simulink model "PHIL_testing"  (R2023b)
settings: Solver=ode4  StartTime=0.0  StopTime=inf  FixedStep=Ts  RelTol=1e-3
PostLoadFcn:
  | init;
InitFcn:
  | init;
values from neighbouring files (symbols this model uses):
  CURRENT_INPUT_OFFSET_PHA = 0    [init.m]
  CURRENT_INPUT_OFFSET_PHB = 0    [init.m]
  CURRENT_INPUT_OFFSET_PHC = 0    [init.m]
  CURRENT_INPUT_SCALE_PHA = 30    [init.m]
  CURRENT_INPUT_SCALE_PHB = 30    [init.m]
  CURRENT_INPUT_SCALE_PHC = 30    [init.m]
  ENABLE_PHA = 1    [init.m]
  ENABLE_PHB = 1    [init.m]
  ENABLE_PHC = 1    [init.m]
  FNOM = 60.0    (= 60)    [init.m]
  FREQUENCY = 60.0    (= 60)    [init.m]
  FREQUENCY_MAX_LIMIT = 66.0    (= 66)    [init.m]
  FREQUENCY_MIN_LIMIT = 56.0    (= 56)    [init.m]
  FRT_CONDITION = [1 1 1 0 ]    [init.m]
  FRT_END_TIMING = [0.2 0.3 0.4 0.5]    [init.m]
  FRT_START_TIMING = [0.1 0.2 0.3 0.4]    [init.m]
  FRT_VALUES = [59.0 56.0 55.0 33.0]    [init.m]
  MODE = 1    [init.m]
  PCRT_CONDITION = [ 0    1     0     2     0     3      0      4      0      4      0   ]    [init.m]
  PCRT_END_TIMING = [30.0 30.32 60.32 60.64 90.64 90.96 120.96 175.96 205.96 260.96 290.96]    [init.m]
  PCRT_START_TIMING = [ 0.0 30.0  30.32 60.32 60.64 90.64  90.96 120.96 175.96 205.96 260.96]    [init.m]
  PCRT_VALUES = [ 0.0 60.0   0.0  60.0   0.0  60.0    0.0   20.0    0.0  340.0    0.0 ]    [init.m]
  PHASE = [0.0 -120.0 120.0]    [init.m]
  PHNOM = [0 -120 120]    [init.m]
  Pnom = 5e3    (= 5000)    [init.m]
  RMS_ENABLE = 0    [init.m]
  ROCOF_ENABLE = 0    [init.m]
  ROCOF_INIT = 60    [init.m]
  ROCOF_VALUE = 3    [init.m]
  ROCOM_ENABLE = 1    [init.m]
  ROCOM_END_TIME = 100    [init.m]
  ROCOM_INIT = 1    [init.m]
  ROCOM_START_TIME = 0    [init.m]
  ROCOM_VALUE = 13.8    [init.m]
  Srated = 5e3    (= 5000)    [init.m]
  Ts = 40e-6    (= 4e-05)    [init.m]
  VNOM = 1.0    (= 1)    [init.m]
  VOLT_INPUT_OFFSET_PHA = 0    [init.m]
  VOLT_INPUT_OFFSET_PHB = 0    [init.m]
  VOLT_INPUT_OFFSET_PHC = 0    [init.m]
  VOLT_INPUT_SCALE_PHA = 100    [init.m]
  VOLT_INPUT_SCALE_PHB = 100    [init.m]
  VOLT_INPUT_SCALE_PHC = 100    [init.m]
  VOLT_OUTPUT_SCALE_PHA = 5.6    [init.m]
  VOLT_OUTPUT_SCALE_PHB = 5.6    [init.m]
  VOLT_OUTPUT_SCALE_PHC = 5.6    [init.m]
  VOLTAGE = [1.0 1.0 1.0]    [init.m]
  VOLTAGE_MAX_LIMIT = 1.1    [init.m]
  VOLTAGE_MIN_LIMIT = 0.0    (= 0)    [init.m]
  VRT_CONDITION = [0 1 0 1 0 1 0 1 -1 -1 -1 -1 -1 -1 -1 -1 -1 -1 -1 -1]+1    [init.m]
  VRT_END_TIMING = [0.2 0.3 0.4 0.5 0.6 0.7 0.8 0.9 1 1.1 1.2 1.3 1.4 1.5 1.6 1.7 1.8 1.9 2 2.1]    [init.m]
  VRT_PHA_ENABLE = 0    [init.m]
  VRT_PHB_ENABLE = 0    [init.m]
  VRT_PHC_ENABLE = 0    [init.m]
  VRT_START_TIMING = [0.1 0.2 0.3 0.4 0.5 0.6 0.7 0.8 0.9 1 0.1 0.2 0.3 0.4 0.5 0.6 0.7 0.8 0.9 1]    [init.m]
  VRT_VALUES = [1.2 0.94 0 0.5 0.7 0.88 0.94 0.88 0.94 1.1 1.2 0.94 0 0.5 0.7 0.88 0.94 0.88 0.94 1.1]    [init.m]
  WAV_ENABLE = 1    [init.m]
undefined symbols (not defined in the file or in its folder): another_event_name, DiscIntNeverNeededParam, EX, magnitude, my_event_name, TE0741_4, TwoSSS_AIO_CPWM
libraries: simulink x14, rtlab x6, simulink_extras x6, spsRMSLib x6, rtio_opalrt_common x4, eePowerMeasurement x3, rtio_opalrt_ml605ex1 x2, spsPLL3phLib x1, spspowerguiLib x1
(part 2 of 2)

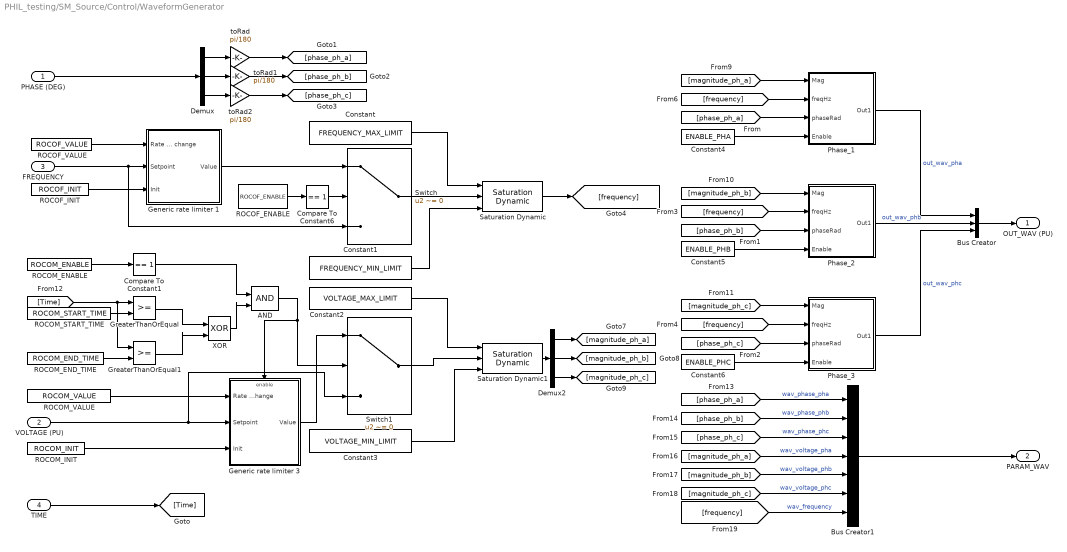
== system PHIL_testing/SM_Source/Control/WaveformGenerator ==
  PHASE (DEG) : Inport
  VOLTAGE (PU) : Inport  Port=2
  FREQUENCY : Inport  Port=3
  TIME : Inport  Port=4
  AND : Logic  IconShape=distinctive  AllPortsSameDT=off  OutDataTypeStr=boolean
  Bus Creator : BusCreator  Inputs=3
  Bus Creator1 : BusCreator  Inputs=7
  Compare To Constant1 : simulink/Logic and Bit Operations/Compare To Constant  relop===  const=1  OutDataTypeStr=boolean
  Compare To Constant6 : simulink/Logic and Bit Operations/Compare To Constant  relop===  const=1  OutDataTypeStr=boolean
  Constant : Constant  Value=FREQUENCY_MAX_LIMIT
  Constant1 : Constant  Value=FREQUENCY_MIN_LIMIT
  Constant2 : Constant  Value=VOLTAGE_MAX_LIMIT
  Constant3 : Constant  Value=VOLTAGE_MIN_LIMIT
  Constant4 : Constant  Value=ENABLE_PHA
  Constant5 : Constant  Value=ENABLE_PHB
  Constant6 : Constant  Value=ENABLE_PHC
  Demux : Demux  Outputs=3
  Demux2 : Demux  Outputs=3
  Generic rate limiter 1 : Subsystem
  Generic rate limiter 3 : Subsystem
  GreaterThanOrEqual : RelationalOperator  OutDataTypeStr=boolean  RndMeth=Simplest  InputSameDT=off
  GreaterThanOrEqual1 : RelationalOperator  OutDataTypeStr=boolean  RndMeth=Simplest  InputSameDT=off
  Phase_1 : Subsystem
  Phase_2 : Subsystem
  Phase_3 : Subsystem
  ROCOF_ENABLE : Constant  Value=ROCOF_ENABLE
  ROCOF_INIT : Constant  Value=ROCOF_INIT
  ROCOF_VALUE : Constant  Value=ROCOF_VALUE
  ROCOM_ENABLE : Constant  Value=ROCOM_ENABLE
  ROCOM_END_TIME : Constant  Value=ROCOM_END_TIME
  ROCOM_INIT : Constant  Value=ROCOM_INIT
  ROCOM_START_TIME : Constant  Value=ROCOM_START_TIME
  ROCOM_VALUE : Constant  Value=ROCOM_VALUE
  Saturation Dynamic : simulink/Discontinuities/Saturation Dynamic  OutMin=[]  OutMax=[]  OutDataTypeStr=Inherit: Same as second input  OutDataType=fixdt(1, 16)  OutScaling=2^-10  DoSatur=off
  Saturation Dynamic1 : simulink/Discontinuities/Saturation Dynamic  OutMin=[]  OutMax=[]  OutDataTypeStr=Inherit: Same as second input  OutDataType=fixdt(1, 16)  OutScaling=2^-10  DoSatur=off
  Switch : Switch  Criteria=u2 ~= 0  SaturateOnIntegerOverflow=off  InputSameDT=off
  Switch1 : Switch  Criteria=u2 ~= 0  SaturateOnIntegerOverflow=off  InputSameDT=off
  XOR : Logic  Operator=XOR  IconShape=distinctive  AllPortsSameDT=off  OutDataTypeStr=boolean
  toRad : Gain  Gain=pi/180
  toRad1 : Gain  Gain=pi/180
  toRad2 : Gain  Gain=pi/180
  OUT_WAV (PU) : Outport
  PARAM_WAV : Outport  Port=2
  wires:
  VOLTAGE (PU)/1 -> Generic rate limiter 3/2("Setpoint "), Switch1/3
  PHASE (DEG)/1 -> Demux/1
  Demux/1 -> toRad/1
  Demux/2 -> toRad1/1
  Demux/3 -> toRad2/1
  [phase_ph_a] -> Phase_1/3(phaseRad)
  [phase_ph_b] -> Phase_2/3(phaseRad)
  [phase_ph_c] -> Phase_3/3(phaseRad)
  Generic rate limiter 1/1(Value) -> Switch/1
  FREQUENCY/1 -> Switch/3, Generic rate limiter 1/2("Setpoint ")
  ROCOF_VALUE/1 -> Generic rate limiter 1/1(Rate of change)
  ROCOF_INIT/1 -> Generic rate limiter 1/3(Init)
  ROCOF_ENABLE/1 -> Compare To Constant6/1
  Compare To Constant6/1 -> Switch/2
  ROCOM_VALUE/1 -> Generic rate limiter 3/1(Rate of change)
  ROCOM_INIT/1 -> Generic rate limiter 3/3(Init)
  [frequency] -> Phase_1/2(freqHz)
  [frequency] -> Phase_2/2(freqHz)
  Demux2/1 -> [magnitude_ph_a]
  Demux2/2 -> [magnitude_ph_b]
  Demux2/3 -> [magnitude_ph_c]
  [magnitude_ph_a] -> Phase_1/1(Mag)
  [magnitude_ph_b] -> Phase_2/1(Mag)
  [magnitude_ph_c] -> Phase_3/1(Mag)
  [Time] -> GreaterThanOrEqual1/1, GreaterThanOrEqual/1
  ROCOM_START_TIME/1 -> GreaterThanOrEqual/2
  ROCOM_END_TIME/1 -> GreaterThanOrEqual1/2
  GreaterThanOrEqual/1 -> XOR/1
  GreaterThanOrEqual1/1 -> XOR/2
  Switch1/1 -> Saturation Dynamic1/2
  Generic rate limiter 3/1(Value) -> Switch1/1
  AND/1 -> Switch1/2, Generic rate limiter 3/Enable
  XOR/1 -> AND/2
  Compare To Constant1/1 -> AND/1
  ROCOM_ENABLE/1 -> Compare To Constant1/1
  Switch/1 -> Saturation Dynamic/2
  TIME/1 -> [Time]
  Phase_1/1(Out1) -> Bus Creator/1  "out_wav_pha"
  Phase_2/1(Out1) -> Bus Creator/2  "out_wav_phb"
  Phase_3/1(Out1) -> Bus Creator/3  "out_wav_phc"
  Bus Creator/1 -> OUT_WAV (PU)/1
  [phase_ph_a] -> Bus Creator1/1  "wav_phase_pha"
  [phase_ph_b] -> Bus Creator1/2  "wav_phase_phb"
  [phase_ph_c] -> Bus Creator1/3  "wav_phase_phc"
  [magnitude_ph_a] -> Bus Creator1/4  "wav_voltage_pha"
  [magnitude_ph_b] -> Bus Creator1/5  "wav_voltage_phb"
  [magnitude_ph_c] -> Bus Creator1/6  "wav_voltage_phc"
  [frequency] -> Bus Creator1/7  "wav_frequency"
  Bus Creator1/1 -> PARAM_WAV/1
  Saturation Dynamic/1 -> [frequency]
  Saturation Dynamic1/1 -> Demux2/1
  Constant/1 -> Saturation Dynamic/1
  Constant1/1 -> Saturation Dynamic/3
  Constant2/1 -> Saturation Dynamic1/1
  Constant3/1 -> Saturation Dynamic1/3
  toRad/1 -> [phase_ph_a]
  toRad1/1 -> [phase_ph_b]
  toRad2/1 -> [phase_ph_c]
  Constant4/1 -> Phase_1/4(Enable)
  Constant5/1 -> Phase_2/4(Enable)
  [frequency] -> Phase_3/2(freqHz)
  Constant6/1 -> Phase_3/4(Enable)

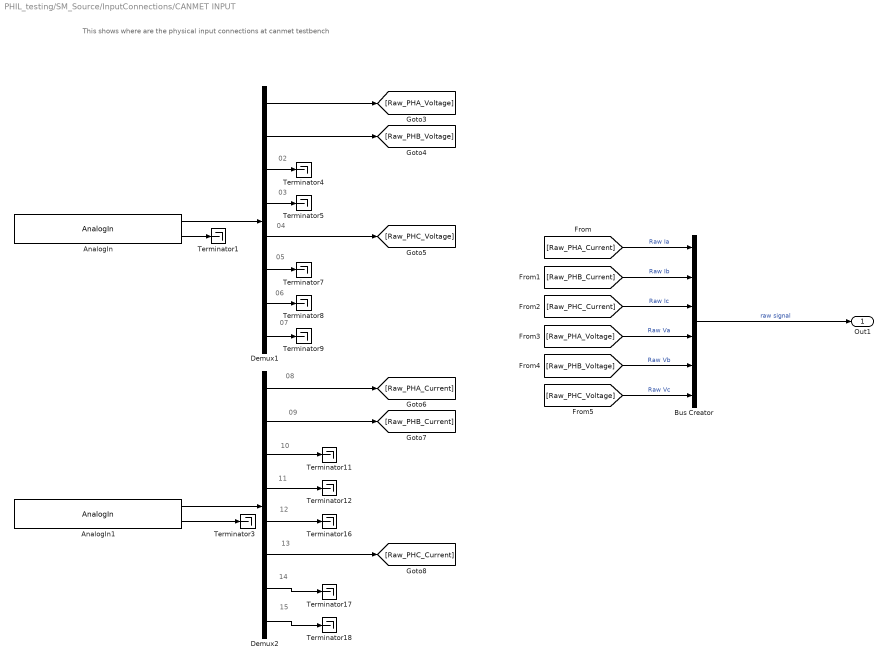
== system PHIL_testing/SM_Source/InputConnections/CANMET INPUT ==
  note: This shows where are the physical input connections at canmet testbench
  note: 10
  note: 08
  note: 03
  note: 04
  note: 15
  note: 12
  note: 09
  note: 06
  note: 11
  note: 07
  note: 05
  note: 02
  note: 13
  note: 14
  AnalogIn : rtio_opalrt_common/AnalogIn  CtrlName='OpCtrl'  portNb=7  FcnNos=Slot 6 Module A Subsection 1  size=16  maxcount=8  count=8  numchan=8  sampleTime=0
      settings: AttributesFormatString=%<CtrlName>  SourceProductName=RT-LAB I/O
  AnalogIn1 : rtio_opalrt_common/AnalogIn  CtrlName='OpCtrl'  portNb=8  FcnNos=Slot 6 Module A Subsection 2  size=16  maxcount=8  count=8  numchan=8  sampleTime=0
      settings: AttributesFormatString=%<CtrlName>  SourceProductName=RT-LAB I/O
  Bus Creator : BusCreator  Inputs=6
  Demux1 : Demux  Outputs=8
  Demux2 : Demux  Outputs=8
  Terminator{1,3..5,7..9,11..12,16..18} (12 alike) : Terminator
  Out1 : Outport  VectorParamsAs1DForOutWhenUnconnected=off
  wires:
  AnalogIn/2 -> Terminator1/1
  AnalogIn1/2 -> Terminator3/1
  AnalogIn/1 -> Demux1/1
  Demux1/4 -> Terminator5/1
  Demux1/7 -> Terminator8/1
  Demux1/6 -> Terminator7/1
  Demux1/8 -> Terminator9/1
  Demux1/3 -> Terminator4/1
  AnalogIn1/1 -> Demux2/1
  Demux2/4 -> Terminator12/1
  Demux2/3 -> Terminator11/1
  Demux2/7 -> Terminator17/1
  Demux2/8 -> Terminator18/1
  Demux2/1 -> [Raw_PHA_Current]
  Demux2/2 -> [Raw_PHB_Current]
  Demux1/5 -> [Raw_PHC_Voltage]
  Demux1/1 -> [Raw_PHA_Voltage]
  Demux1/2 -> [Raw_PHB_Voltage]
  [Raw_PHC_Current] -> Bus Creator/3  "Raw Ic"
  [Raw_PHB_Current] -> Bus Creator/2  "Raw Ib"
  [Raw_PHA_Current] -> Bus Creator/1  "Raw Ia"
  [Raw_PHA_Voltage] -> Bus Creator/4  "Raw Va"
  [Raw_PHB_Voltage] -> Bus Creator/5  "Raw Vb"
  [Raw_PHC_Voltage] -> Bus Creator/6  "Raw Vc"
  Bus Creator/1 -> Out1/1  "raw signal"
  Demux2/5 -> Terminator16/1
  Demux2/6 -> [Raw_PHC_Current]

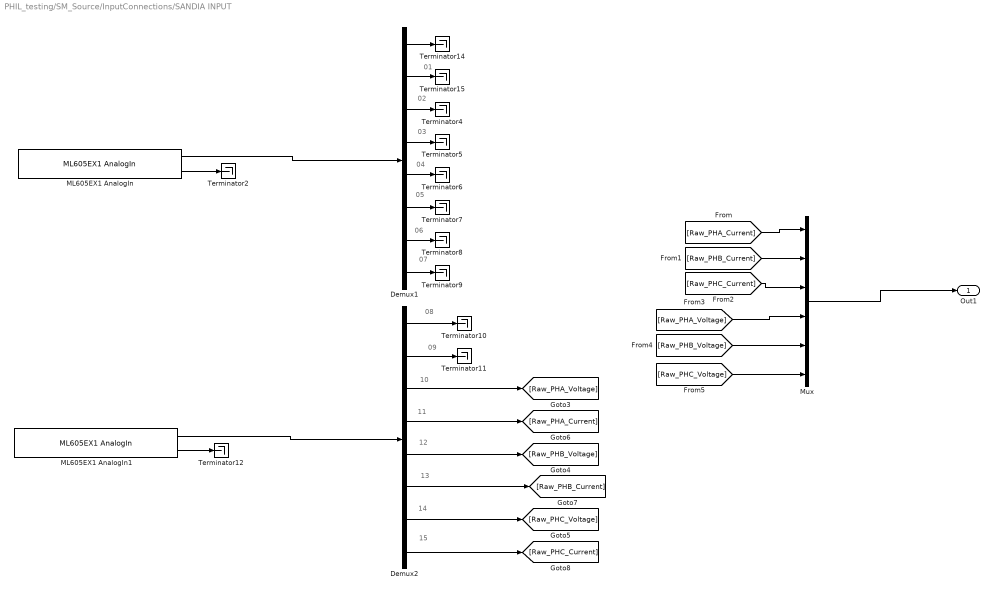
== system PHIL_testing/SM_Source/InputConnections/SANDIA INPUT ==
  note: 11
  note: 14
  note: 09
  note: 04
  note: 06
  note: 05
  note: 02
  note: 12
  note: 03
  note: 13
  note: 15
  note: 07
  note: 08
  note: 10
  note: 01
  Demux1 : Demux  Outputs=8
  Demux2 : Demux  Outputs=8
  ML605EX1 AnalogIn : rtio_opalrt_ml605ex1/ML605EX1 AnalogIn  CtrlName='ML605EX1 Ctrl'  portNb=1  FcnNos=Slot 0 Module X Subsection 0  size=0  maxcount=0  count=8  numchan=8  sampleTime=0
      settings: AttributesFormatString=%<CtrlName>  SourceProductName=RT-LAB I/O
  ML605EX1 AnalogIn1 : rtio_opalrt_ml605ex1/ML605EX1 AnalogIn  CtrlName='ML605EX1 Ctrl'  portNb=2  FcnNos=Slot 0 Module X Subsection 0  size=0  maxcount=0  count=8  numchan=8  sampleTime=0
      settings: AttributesFormatString=%<CtrlName>  SourceProductName=RT-LAB I/O
  Mux : Mux  Inputs=6
  Terminator{2,4..12,14..15} (12 alike) : Terminator
  Out1 : Outport  VectorParamsAs1DForOutWhenUnconnected=off
  wires:
  ML605EX1 AnalogIn1/2 -> Terminator12/1
  ML605EX1 AnalogIn/2 -> Terminator2/1
  Demux2/2 -> Terminator11/1
  Demux1/1 -> Terminator14/1
  Demux2/1 -> Terminator10/1
  Demux1/8 -> Terminator9/1
  Demux1/3 -> Terminator4/1
  Demux1/5 -> Terminator6/1
  Demux1/6 -> Terminator7/1
  Demux1/7 -> Terminator8/1
  Demux1/2 -> Terminator15/1
  Demux1/4 -> Terminator5/1
  ML605EX1 AnalogIn/1 -> Demux1/1
  ML605EX1 AnalogIn1/1 -> Demux2/1
  Demux2/6 -> [Raw_PHB_Current]
  Demux2/7 -> [Raw_PHC_Voltage]
  Demux2/8 -> [Raw_PHC_Current]
  Demux2/3 -> [Raw_PHA_Voltage]
  Demux2/5 -> [Raw_PHB_Voltage]
  Demux2/4 -> [Raw_PHA_Current]
  Mux/1 -> Out1/1
  [Raw_PHC_Current] -> Mux/3
  [Raw_PHA_Voltage] -> Mux/4
  [Raw_PHC_Voltage] -> Mux/6
  [Raw_PHA_Current] -> Mux/1
  [Raw_PHB_Voltage] -> Mux/5
  [Raw_PHB_Current] -> Mux/2

== system PHIL_testing/SM_Source/Control/DataAcquisitionSystem/Subsystem ==
  In1 : Inport
  Enable : EnablePort
  FILE_LIMIT : Gain
  FILE_STATUS : Gain
  OpWriteFile : rtlab/DataLogging/OpWriteFile  Static_File=on  varname=Data  Filename=Data.mat  rtpath='./'  nrtpath='.\'  Acq_Group=27  file_size=1e+8  write_offline=off  Sim_Mode=off  Nb_Samples=500  Buffer_size=200000
      settings: SourceProductName=RT-LAB  Decimation=25
  Terminator : Terminator
  Terminator1 : Terminator
  wires:
  OpWriteFile/1 -> FILE_LIMIT/1
  FILE_LIMIT/1 -> Terminator/1
  OpWriteFile/2 -> FILE_STATUS/1
  FILE_STATUS/1 -> Terminator1/1
  In1/1 -> OpWriteFile/1

== system PHIL_testing/SM_Source/Control/DataAcquisitionSystem/Subsystem1 ==
  In1 : Inport
  Enable : EnablePort
  FILE_LIMIT : Gain
  FILE_STATUS : Gain
  OpWriteFile : rtlab/DataLogging/OpWriteFile  Static_File=on  varname=Data  Filename=WAV.mat  rtpath='./'  nrtpath='.\'  Acq_Group=28  file_size=3e+8  write_offline=off  Sim_Mode=off  Nb_Samples=1000  Buffer_size=200000
      settings: SourceProductName=RT-LAB  Decimation=4
  Terminator : Terminator
  Terminator1 : Terminator
  wires:
  In1/1 -> OpWriteFile/1
  FILE_STATUS/1 -> Terminator1/1
  OpWriteFile/2 -> FILE_STATUS/1
  FILE_LIMIT/1 -> Terminator/1
  OpWriteFile/1 -> FILE_LIMIT/1

== system PHIL_testing/SM_Source/Control/SignalConditioning/Subsystem ==
  P : Inport
  Q : Inport  Port=2
  Divide : Product  Inputs=*/
  Math Function6 : Math  Operator=hypot  SignedPower=on
  Saturation : Saturate  UpperLimit=1.1  LowerLimit=0
  PF : Outport  VectorParamsAs1DForOutWhenUnconnected=off
  wires:
  Divide/1 -> Saturation/1
  P/1 -> Divide/1, Math Function6/1
  Q/1 -> Math Function6/2
  Math Function6/1 -> Divide/2
  Saturation/1 -> PF/1

== system PHIL_testing/SM_Source/Control/SignalConditioning/Subsystem1 ==
  P : Inport
  Q : Inport  Port=2
  Divide : Product  Inputs=*/
  Math Function6 : Math  Operator=hypot  SignedPower=on
  Saturation : Saturate  UpperLimit=1.1  LowerLimit=0
  PF : Outport  VectorParamsAs1DForOutWhenUnconnected=off
  wires:
  Saturation/1 -> PF/1
  Math Function6/1 -> Divide/2
  Q/1 -> Math Function6/2
  P/1 -> Math Function6/1, Divide/1
  Divide/1 -> Saturation/1

== system PHIL_testing/SM_Source/Control/SignalConditioning/Subsystem2 ==
  P : Inport
  Q : Inport  Port=2
  Divide : Product  Inputs=*/
  Math Function6 : Math  Operator=hypot  SignedPower=on
  Saturation : Saturate  UpperLimit=1.1  LowerLimit=0
  PF : Outport  VectorParamsAs1DForOutWhenUnconnected=off
  wires:
  Divide/1 -> Saturation/1
  P/1 -> Divide/1, Math Function6/1
  Q/1 -> Math Function6/2
  Math Function6/1 -> Divide/2
  Saturation/1 -> PF/1

== system PHIL_testing/SM_Source/Control/WaveformGenerator/Generic rate limiter 1 ==
  Rate of change : Inport
  "Setpoint " : Inport  Port=2
  Init : Inport  Port=3
  Add1 : Sum  Inputs=+-
  Add2 : Sum
  Gain : Gain  Gain=-1
  Rate Limiter Dynamic : simulink/Discontinuities/Rate Limiter Dynamic
  Value : Outport  VectorParamsAs1DForOutWhenUnconnected=off
  wires:
  Rate Limiter Dynamic/1 -> Add2/1  "Freq"
  Add2/1 -> Value/1  "Freq"
  Gain/1 -> Rate Limiter Dynamic/3
  Add1/1 -> Rate Limiter Dynamic/2
  "Setpoint "/1 -> Add1/1
  Rate of change/1 -> Gain/1, Rate Limiter Dynamic/1
  Init/1 -> Add1/2, Add2/2

== system PHIL_testing/SM_Source/Control/WaveformGenerator/Generic rate limiter 3 ==
  Rate of change : Inport
  "Setpoint " : Inport  Port=2
  Init : Inport  Port=3
  Enable : EnablePort
  Add1 : Sum  Inputs=+-
  Add2 : Sum
  Gain : Gain  Gain=-1
  Rate Limiter Dynamic : simulink/Discontinuities/Rate Limiter Dynamic
  Value : Outport  VectorParamsAs1DForOutWhenUnconnected=off
  wires:
  Init/1 -> Add2/2, Add1/2
  Rate of change/1 -> Rate Limiter Dynamic/1, Gain/1
  "Setpoint "/1 -> Add1/1
  Add1/1 -> Rate Limiter Dynamic/2
  Gain/1 -> Rate Limiter Dynamic/3
  Add2/1 -> Value/1
  Rate Limiter Dynamic/1 -> Add2/1

== system PHIL_testing/SM_Source/Control/WaveformGenerator/Phase_1 ==
  Mag : Inport
  freqHz : Inport  Port=2
  phaseRad : Inport  Port=3
  Enable : Inport  Port=4
  2pi : Gain  Gain=2*pi
  Add : Sum
  Constant : Constant  Value=0
  Discrete-Time Integrator : DiscreteIntegrator  SampleTime=Ts  ICPrevOutput=DiscIntNeverNeededParam  ICPrevScaledInput=DiscIntNeverNeededParam
  Product1 : Product
  Scope : Scope
  Switch : Switch  Criteria=u2 > Threshold  SaturateOnIntegerOverflow=off  InputSameDT=off
  Trigonometric Function : Trigonometry  Operator=cos  OutputSignalType=real
  Out1 : Outport  VectorParamsAs1DForOutWhenUnconnected=off
  wires:
  Mag/1 -> Product1/1
  Trigonometric Function/1 -> Scope/1, Product1/2
  freqHz/1 -> 2pi/1  "f"
  phaseRad/1 -> Add/2  "phi"
  Product1/1 -> Switch/1
  2pi/1 -> Discrete-Time Integrator/1  "w"
  Discrete-Time Integrator/1 -> Add/1  "wt"
  Add/1 -> Trigonometric Function/1  "wt+phi"
  Enable/1 -> Switch/2
  Switch/1 -> Out1/1
  Constant/1 -> Switch/3

== system PHIL_testing/SM_Source/Control/WaveformGenerator/Phase_2 ==
  Mag : Inport
  freqHz : Inport  Port=2
  phaseRad : Inport  Port=3
  Enable : Inport  Port=4
  2pi : Gain  Gain=2*pi
  Add : Sum
  Constant : Constant  Value=0
  Discrete-Time Integrator : DiscreteIntegrator  SampleTime=Ts  ICPrevOutput=DiscIntNeverNeededParam  ICPrevScaledInput=DiscIntNeverNeededParam
  Product1 : Product
  Scope : Scope
  Switch : Switch  Criteria=u2 > Threshold  SaturateOnIntegerOverflow=off  InputSameDT=off
  Trigonometric Function : Trigonometry  Operator=cos  OutputSignalType=real
  Out1 : Outport  VectorParamsAs1DForOutWhenUnconnected=off
  wires:
  Constant/1 -> Switch/3
  Switch/1 -> Out1/1
  Enable/1 -> Switch/2
  Add/1 -> Trigonometric Function/1  "wt+phi"
  Discrete-Time Integrator/1 -> Add/1  "wt"
  2pi/1 -> Discrete-Time Integrator/1  "w"
  Product1/1 -> Switch/1
  phaseRad/1 -> Add/2  "phi"
  freqHz/1 -> 2pi/1  "f"
  Trigonometric Function/1 -> Product1/2, Scope/1
  Mag/1 -> Product1/1

== system PHIL_testing/SM_Source/Control/WaveformGenerator/Phase_3 ==
  Mag : Inport
  freqHz : Inport  Port=2
  phaseRad : Inport  Port=3
  Enable : Inport  Port=4
  2pi : Gain  Gain=2*pi
  Add : Sum
  Constant : Constant  Value=0
  Discrete-Time Integrator : DiscreteIntegrator  SampleTime=Ts  ICPrevOutput=DiscIntNeverNeededParam  ICPrevScaledInput=DiscIntNeverNeededParam
  Product1 : Product
  Scope : Scope
  Switch : Switch  Criteria=u2 > Threshold  SaturateOnIntegerOverflow=off  InputSameDT=off
  Trigonometric Function : Trigonometry  Operator=cos  OutputSignalType=real
  Out1 : Outport  VectorParamsAs1DForOutWhenUnconnected=off
  wires:
  Mag/1 -> Product1/1
  Trigonometric Function/1 -> Scope/1, Product1/2
  freqHz/1 -> 2pi/1  "f"
  phaseRad/1 -> Add/2  "phi"
  Product1/1 -> Switch/1
  2pi/1 -> Discrete-Time Integrator/1  "w"
  Discrete-Time Integrator/1 -> Add/1  "wt"
  Add/1 -> Trigonometric Function/1  "wt+phi"
  Enable/1 -> Switch/2
  Switch/1 -> Out1/1
  Constant/1 -> Switch/3

== matlab function PHIL_testing/SM_Source/Control/FRT/MATLAB Function1 ==
  settings: updateMethod=DISCRETE
  data: TIME input; COMMAND output; CONDITIONS input; START_TIMING input; END_TIMING input; VALUES input; TRIGGER output; TEST_CONDITION output; COMPLETED output; NOMINAL input
function [COMMAND, TRIGGER, TEST_CONDITION, COMPLETED] = disturbances_logic(TIME,CONDITIONS,START_TIMING,END_TIMING,VALUES, NOMINAL)

% all actions are condition actions and 
% outputs are function of state and input 
persistent current_value;
persistent current_state;
persistent current_trigger;
persistent index;
persistent current_test_condition;

% define states
START = 0;
CHECK_TIMING = 1;
NEXT_INDEX = 2;
LAST_INDEX = 3;
COMPLETED_SEQUENCE = 4;
% Define useful variables

% Make sure variables are initialize
if isempty(current_value)
    current_value = NOMINAL; 
end
if isempty(current_state)
    current_state = START; 
end
if isempty(current_trigger)
    current_trigger = 0;   
end
if isempty(index)
    index = 1;   
end
if isempty(current_test_condition)
    current_test_condition = 0;   
end
% Simple state machine to handle iteration base on time
switch (current_state) 
    case START,
        % value of output 'command' depends both on state and inputs
        if (TIME > START_TIMING(index))
            current_state = CHECK_TIMING;
        else
            current_state = START;
            % Start at nominal
            current_value = NOMINAL; 

        end
    case CHECK_TIMING,
        % value of output 'command' depends both on state and inputs
        if (TIME>END_TIMING(index))
            current_state = NEXT_INDEX;
        else
            current_state = CHECK_TIMING;
            current_value = VALUES(index);
            current_test_condition = CONDITIONS(index)
            current_trigger = 1;

        end
    case NEXT_INDEX,
        % value of output 'command' depends both on state and inputs
        index = index + 1 
        if(CONDITIONS(index + 1) == 0)
            current_state = LAST_INDEX;
        else
            current_state = CHECK_TIMING;
        end
    case LAST_INDEX,
        if (TIME>END_TIMING(index))
            current_state = COMPLETED_SEQUENCE;
        else
            current_state = LAST_INDEX;
            current_value = VALUES(index);
            current_test_condition = CONDITIONS(index)

        end
    case COMPLETED_SEQUENCE,
        % Going back to nominal, in case other sequences needed
        current_state = COMPLETED_SEQUENCE;
        current_trigger = 0;
        current_value = NOMINAL; 
        current_test_condition = 0

end
TEST_CONDITION = current_test_condition;
COMMAND = current_value;
TRIGGER = current_trigger;

if (current_state == COMPLETED_SEQUENCE)
    COMPLETED = 1;
else
    COMPLETED = 0;
end

== matlab function PHIL_testing/SM_Source/Control/PCRT/MATLAB Function1 ==
  settings: updateMethod=DISCRETE
  data: TIME input; COMMAND output; CONDITIONS input; START_TIMING input; END_TIMING input; VALUES input; TRIGGER output; TEST_CONDITION output; COMPLETED output; NOMINAL input
function [COMMAND, TRIGGER, TEST_CONDITION, COMPLETED] = disturbances_logic(TIME,CONDITIONS,START_TIMING,END_TIMING,VALUES, NOMINAL)

% all actions are condition actions and 
% outputs are function of state and input 
persistent current_value;
persistent current_state;
persistent current_trigger;
persistent index;
persistent current_test_condition;

% define states
START = 0;
CHECK_TIMING = 1;
NEXT_INDEX = 2;
LAST_INDEX = 3;
COMPLETED_SEQUENCE = 4;
% Define useful variables

% Make sure variables are initialize
if isempty(current_value)
    current_value = NOMINAL; 
end
if isempty(current_state)
    current_state = START; 
end
if isempty(current_trigger)
    current_trigger = 0;   
end
if isempty(index)
    index = 1;   
end
if isempty(current_test_condition)
    current_test_condition = 0;   
end
% Simple state machine to handle iteration base on time
switch (current_state) 
    case START,
        % value of output 'command' depends both on state and inputs
        if (TIME > START_TIMING(index))
            current_state = CHECK_TIMING;
        else
            current_state = START;
            % Start at nominal
            current_value = NOMINAL; 

        end
    case CHECK_TIMING,
        % value of output 'command' depends both on state and inputs
        if (TIME>END_TIMING(index))
            current_state = NEXT_INDEX;
        else
            current_state = CHECK_TIMING;
            current_test_condition = CONDITIONS(index)
            switch (current_test_condition)
                case 1,
                    current_value = NOMINAL;
                case 2,
                    current_value = NOMINAL + [VALUES(index), 0, 0]';
                case 3,
                    current_value = NOMINAL + [0, VALUES(index), 0]';
                case 4,
                    current_value = NOMINAL + [0, 0, VALUES(index)]';
                case 5,
                    current_value = NOMINAL + VALUES(index);
                case 6,
                    current_value = NOMINAL - VALUES(index);
            end
            
            current_trigger = 1;

        end
    case NEXT_INDEX,
        % value of output 'command' depends both on state and inputs
        index = index + 1 
        if(CONDITIONS(index + 1) == 0)
            current_state = LAST_INDEX;
        else
            current_state = CHECK_TIMING;
        end
    case LAST_INDEX,
        if (TIME>END_TIMING(index))
            current_state = COMPLETED_SEQUENCE;
        else
            current_state = LAST_INDEX;
            current_test_condition = CONDITIONS(index)
            switch (current_test_condition)
                case 1,
                    current_value = NOMINAL;
                case 2,
                    current_value = NOMINAL + [VALUES(index), 0, 0]';
                case 3,
                    current_value = NOMINAL + [0, VALUES(index), 0]';
                case 4,
                    current_value = NOMINAL + [0, 0, VALUES(index)]';
                case 5,
                    current_value = NOMINAL + VALUES(index);
                 case 6,
                    current_value = NOMINAL - VALUES(index);
            end
        end
    case COMPLETED_SEQUENCE,
        % Going back to nominal, in case other sequences needed
        current_state = COMPLETED_SEQUENCE;
        current_trigger = 0;
        current_value = NOMINAL; 
        current_test_condition = 0

end
TEST_CONDITION = current_test_condition;
COMMAND = current_value;
TRIGGER = current_trigger;

if (current_state == COMPLETED_SEQUENCE)
    COMPLETED = 1;
else
    COMPLETED = 0;
end

== matlab function PHIL_testing/SM_Source/Control/VRT/MATLAB Function1 ==
  settings: updateMethod=DISCRETE
  data: TIME input; COMMAND output; CONDITIONS input; START_TIMING input; END_TIMING input; VALUES input; TRIGGER output; TEST_CONDITION output; COMPLETED output; NOMINAL input
function [COMMAND, TRIGGER, TEST_CONDITION, COMPLETED] = disturbances_logic(TIME,CONDITIONS,START_TIMING,END_TIMING,VALUES, NOMINAL)

% all actions are condition actions and 
% outputs are function of state and input 
persistent current_value;
persistent current_state;
persistent current_trigger;
persistent index;
persistent current_test_condition;

% define states
START = 0;
CHECK_TIMING = 1;
NEXT_INDEX = 2;
LAST_INDEX = 3;
COMPLETED_SEQUENCE = 4;
% Define useful variables

% Make sure variables are initialize
if isempty(current_value)
    current_value = NOMINAL; 
end
if isempty(current_state)
    current_state = START; 
end
if isempty(current_trigger)
    current_trigger = 0;   
end
if isempty(current_test_condition)
    current_test_condition = 0;   
end
if isempty(index)
    index = 1;   
end
% Simple state machine to handle iteration base on time
switch (current_state) 
    case START,
        % value of output 'command' depends both on state and inputs
        if (TIME > START_TIMING(index))
            current_state = CHECK_TIMING;
        else
            current_state = START;
            % Start at nominal
            current_value = NOMINAL; 

        end
    case CHECK_TIMING,
        % value of output 'command' depends both on state and inputs
        if (TIME>END_TIMING(index))
            current_state = NEXT_INDEX;
        else
            current_state = CHECK_TIMING;
            current_value = VALUES(index);
            current_test_condition = CONDITIONS(index)
            current_trigger = 1;

        end
    case NEXT_INDEX,
        % value of output 'command' depends both on state and inputs
        index = index + 1 
        if(CONDITIONS(index + 1) == 0)
            current_state = LAST_INDEX;
        else
            current_state = CHECK_TIMING;
        end
    case LAST_INDEX,
        if (TIME>END_TIMING(index))
            current_state = COMPLETED_SEQUENCE;
        else
            current_state = LAST_INDEX;
            current_value = VALUES(index);
            current_test_condition = CONDITIONS(index)

        end
    case COMPLETED_SEQUENCE,
        % Going back to nominal, in case other sequences needed
        current_state = COMPLETED_SEQUENCE;
        current_trigger = 0;
        current_value = NOMINAL; 
        current_test_condition = 0

end
TEST_CONDITION = current_test_condition;
COMMAND = current_value;
TRIGGER = current_trigger;


if (current_state == COMPLETED_SEQUENCE)
    COMPLETED = 1;
else
    COMPLETED = 0;
end
